simulink model "gm_untitled1"  (R2023a)
settings: Solver=FixedStepAuto  StartTime=0.0  StopTime=5  RelTol=1e-3
settings Model: Creator=Tien  LastModifiedBy=Tien
settings OptimizationCC: BlockReduction=off  ConditionallyExecuteInputs=off
settings DebuggingCC: InheritedTsInSrcMsg=none  ParameterPrecisionLossMsg=none

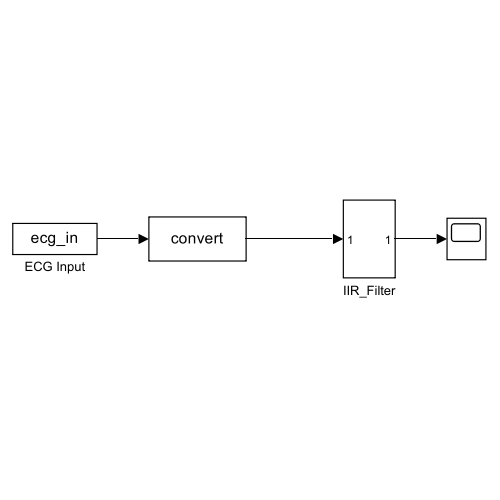
[thumbnail: Simulink's stored preview of the top-level diagram]
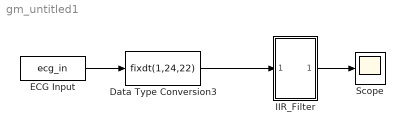
== system gm_untitled1 ==
  Data Type Conversion3 : DataTypeConversion  OutDataTypeStr=fixdt(1,24,22)  RndMeth=Round
  ECG Input : FromWorkspace  VariableName=ecg_in  SampleTime=0.002
  IIR_Filter : Subsystem
  Scope : Scope
  wires:
  IIR_Filter/1(Out1) -> Scope/1
  Data Type Conversion3/1 -> IIR_Filter/1(In1)
  ECG Input/1 -> Data Type Conversion3/1

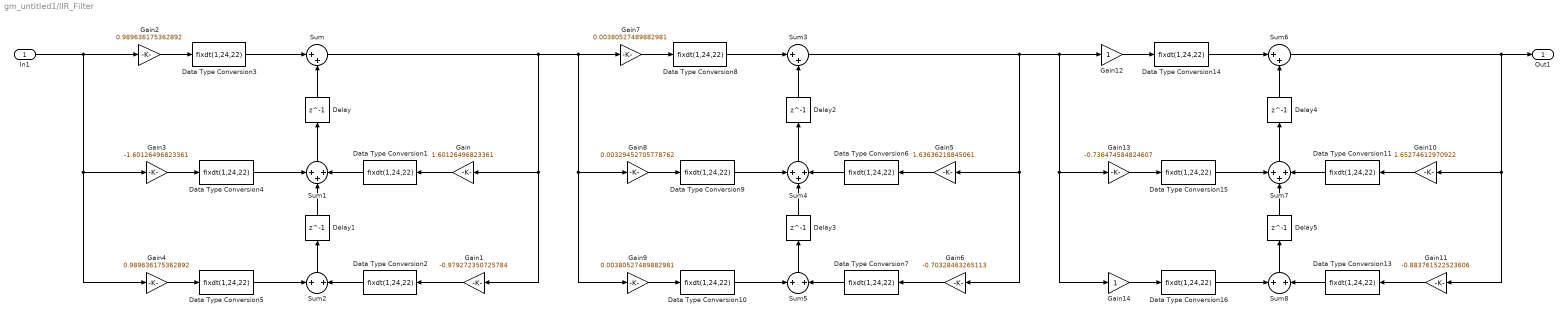
== system gm_untitled1/IIR_Filter ==
  In1 : Inport  OutDataTypeStr=fixdt(1,24,22)
  Data Type Conversion{1..11,13..16} (15 alike) : DataTypeConversion  OutDataTypeStr=fixdt(1,24,22)  RndMeth=Round
  Delay{,1..5} (6 alike) : Delay  DelayLength=1  InitialCondition=0
  Gain : Gain  Gain=1.60126496823361  RndMeth=Round  SaturateOnIntegerOverflow=on
  Gain1 : Gain  Gain=-0.979272350725784
  Gain10 : Gain  Gain=1.65274612970922  RndMeth=Round  SaturateOnIntegerOverflow=on
  Gain11 : Gain  Gain=-0.883761522523606
  Gain12 : Gain  RndMeth=Nearest
  Gain13 : Gain  Gain=-0.736474584824607  RndMeth=Round
  Gain14 : Gain
  Gain2 : Gain  Gain=0.989636175362892  RndMeth=Nearest
  Gain3 : Gain  Gain=-1.60126496823361  RndMeth=Round
  Gain4 : Gain  Gain=0.989636175362892
  Gain5 : Gain  Gain=1.63636218845061  RndMeth=Round  SaturateOnIntegerOverflow=on
  Gain6 : Gain  Gain=-0.70328463265113
  Gain7 : Gain  Gain=0.00380527489882981  RndMeth=Nearest
  Gain8 : Gain  Gain=0.00329452705778762  RndMeth=Round
  Gain9 : Gain  Gain=0.00380527489882981
  Sum : Sum  Inputs=|++  OutDataTypeStr=fixdt(1,40,30)  RndMeth=Round  SaturateOnIntegerOverflow=on
  Sum1 : Sum  Inputs=+++  OutDataTypeStr=fixdt(1,40,30)  RndMeth=Round  SaturateOnIntegerOverflow=on
  Sum2 : Sum  Inputs=+|+  OutDataTypeStr=fixdt(1,40,30)  RndMeth=Round  SaturateOnIntegerOverflow=on
  Sum3 : Sum  Inputs=|++  OutDataTypeStr=fixdt(1,40,30)  RndMeth=Round  SaturateOnIntegerOverflow=on
  Sum4 : Sum  Inputs=+++  OutDataTypeStr=fixdt(1,40,30)  RndMeth=Round  SaturateOnIntegerOverflow=on
  Sum5 : Sum  Inputs=+|+  OutDataTypeStr=fixdt(1,40,30)  RndMeth=Round  SaturateOnIntegerOverflow=on
  Sum6 : Sum  Inputs=|++  OutDataTypeStr=fixdt(1,40,30)  RndMeth=Round  SaturateOnIntegerOverflow=on
  Sum7 : Sum  Inputs=+++  OutDataTypeStr=fixdt(1,40,30)  RndMeth=Round  SaturateOnIntegerOverflow=on
  Sum8 : Sum  Inputs=+|+  OutDataTypeStr=fixdt(1,40,30)  RndMeth=Round  SaturateOnIntegerOverflow=on
  Out1 : Outport  OutDataTypeStr=fixdt(1,40,30)
  wires:
  In1/1 -> Gain2/1, Gain3/1, Gain4/1
  Delay4/1 -> Sum6/2
  Sum3/1 -> Gain5/1, Gain6/1, Gain12/1, Gain13/1, Gain14/1
  Data Type Conversion11/1 -> Sum7/3
  Gain10/1 -> Data Type Conversion11/1
  Data Type Conversion16/1 -> Sum8/1
  Sum7/1 -> Delay4/1
  Data Type Conversion14/1 -> Sum6/1
  Data Type Conversion13/1 -> Sum8/2
  Sum6/1 -> Gain10/1, Gain11/1, Out1/1
  Delay5/1 -> Sum7/2
  Gain12/1 -> Data Type Conversion14/1
  Sum8/1 -> Delay5/1
  Gain14/1 -> Data Type Conversion16/1
  Gain13/1 -> Data Type Conversion15/1
  Data Type Conversion15/1 -> Sum7/1
  Gain11/1 -> Data Type Conversion13/1
  Delay2/1 -> Sum3/2
  Sum/1 -> Gain/1, Gain1/1, Gain7/1, Gain8/1, Gain9/1
  Data Type Conversion6/1 -> Sum4/3
  Gain5/1 -> Data Type Conversion6/1
  Data Type Conversion10/1 -> Sum5/1
  Sum4/1 -> Delay2/1
  Data Type Conversion8/1 -> Sum3/1
  Data Type Conversion7/1 -> Sum5/2
  Delay3/1 -> Sum4/2
  Gain7/1 -> Data Type Conversion8/1
  Sum5/1 -> Delay3/1
  Gain9/1 -> Data Type Conversion10/1
  Gain8/1 -> Data Type Conversion9/1
  Data Type Conversion9/1 -> Sum4/1
  Gain6/1 -> Data Type Conversion7/1
  Data Type Conversion4/1 -> Sum1/1
  Gain3/1 -> Data Type Conversion4/1
  Gain2/1 -> Data Type Conversion3/1
  Sum2/1 -> Delay1/1
  Data Type Conversion2/1 -> Sum2/2
  Gain1/1 -> Data Type Conversion2/1
  Data Type Conversion3/1 -> Sum/1
  Gain/1 -> Data Type Conversion1/1
  Sum1/1 -> Delay/1
  Data Type Conversion1/1 -> Sum1/3
  Delay/1 -> Sum/2
  Data Type Conversion5/1 -> Sum2/1
  Delay1/1 -> Sum1/2
  Gain4/1 -> Data Type Conversion5/1
